simulink model "et_robocon_emer"  (R2014b)
settings: Solver=ode3  SolverMode=SingleTasking  StartTime=0.0  StopTime=10.0  RelTol=1e-3
undefined symbols (not defined in the file): balancerStates_Bus0, Batt, current_mode_status, current_task_operation_status, GYRO, Init_Bus0, K, lightCalib, PHI, R, RM, Th, TRACK_MODE_LIST, W
libraries: legonxtlib x27, ControllersFcns x5, simulink_extras x4, simulink x3, NXTFcns x2, gyro_calibration_algorithm_atomic_sub_chart_library x1, light_sensor_calibration_algorithm_atomic_sub_chart_library x1, plantNXT x1
(part 2 of 2)

== stateflow chart et_robocon_emer/Main Controller/normal_operation_modes.line_following_down ==
  state RampDownDir
    entry:
    StatusLCD(uint16(400));
    des_vel = single(0);
    desired_tail = single(0.0);
    BT_status_out = single(11);
    turningPWM = single(0);
    initFlags.theta = single(1);
    initFlags.gyroReset = single(1);
    Speak;
    during:
    normalizedLight = processLight(sensors.light,lightCalib);
    PWM.tail = tail_controller(sensors.theta_T, desired_tail);
    state Waiting
      entry:
      during:
      StatusLCD(uint16(400));
    state light = processLight(rawLight,lightCalib) [function]
    state cmd = lineTracker(desiredLight,light,trackingPower,battery) [function]
    state StandUp1
      entry:
      StatusLCD(uint16(401));
      initFlags.theta = single(1);
      initFlags.gyroReset = single(1);
    state cmd = balance_ctrl(balancerStates,desired_velocity,battery) [function]
    state Balancing
      state SeesawLogic [parallel]
        settings: executionOrder=2
        state MoveForwardSlowly
          entry:
          Speak;
          StatusLCD(uint16(402));
          des_vel = single(0.0);
          initFlags.theta = single(0);
          initFlags.gyroReset = single(0);
          storedphi = states.phi;
          tix = 1;
          des_vel = single(0.005);
          desired_phi = storedphi;
          thetaentry = states.balancerStates.theta;
          during:
          storedphi = storedphi+states.phi;
          tix = tix+1;
          turningPWM = lineTracker(single(-0.3), normalizedLight, single(1.5), sensors.battery)+...
          single(.5)*phiController(desired_phi,states.phi,sensors.battery);
        state StationnaryBalance
          entry:
          Speak;
          StatusLCD(uint16(403));
          storedphi = single(storedphi/tix);
          %StatusLCD(uint16(single(0.15)));
          des_vel = single(0.01);
          desired_phi = states.phi;
          during:
          des_vel = des_vel+single(0.001)
          turningPWM = lineTracker(single(-0.3), normalizedLight, single(1.5), sensors.battery)+...
          single(.5)*phiController(desired_phi,states.phi,sensors.battery);
          if des_vel > single(0.05)
          des_vel = single(0.05);
          end
        state constspeed
          entry: StatusLCD(uint16(404));
          during:
          turningPWM = phiController(desired_phi,states.phi,sensors.battery);
        state Ramps
          state Ramp2
            entry:
            thetaentry = states.balancerStates.theta;
            Speak;
            desired_phi = storedphi;
            %+single(0.5);
            %storedphi = states.phi;
            tix = 1;
            %Speak;
            StatusLCD(uint16(405));
            des_vel = single(0.03);
            %desired_phi = storedphi;
            during:
            %storedphi = storedphi +states.phi;
            %tix = tix+1;
            %des_vel = single(0.04);
            turningPWM = phiController(desired_phi,states.phi,sensors.battery);
            %turningPWM = lineTracker(single(-0.2),normalizedLight,single(1.5),sensors.battery)+...
            % single(.4)*phiController(desired_phi,states.phi,sensors.battery);
          state TurnLineTrackOn
            entry:
            StatusLCD(uint16(406));
            during:
            turningPWM = lineTracker(single(0.7),normalizedLight,single(1.5),sensors.battery)+...
            single(.5)*phiController(desired_phi,states.phi,sensors.battery);
          state Bridge
            entry:
            thetaentry = states.balancerStates.theta;
            Speak;
            StatusLCD(uint16(407));
            %storedphi = single(storedphi/tix);
            desired_phi  = storedphi;
            during:
            des_vel =single(0.04);
            turningPWM = phiController(desired_phi,states.phi,sensors.battery);
          state Ramp1
            entry:
            thetaentry = states.balancerStates.theta;
            des_vel= single(0.02);
            Speak;
            StatusLCD(uint16(408));
            during:
            during:
            turningPWM = lineTracker(single(0.7),normalizedLight,single(1.5),sensors.battery)+...
            single(.5)*phiController(desired_phi,states.phi,sensors.battery);
          state Land
            entry:
            des_vel= single(0.005);
            Speak;
            StatusLCD(uint16(409));
            during:
            turningPWM = phiController(desired_phi,states.phi,sensors.battery);
          (default) -> RampDownDir.Balancing.SeesawLogic.Ramps.Ramp2
          RampDownDir.Balancing.SeesawLogic.Ramps.Ramp2 -> TurnLineTrackOn : [states.balancerStates.theta>thetaentry + single(1*2*3.14) ]
          TurnLineTrackOn -> RampDownDir.Balancing.SeesawLogic.Ramps.Bridge : [states.balancerStates.theta>thetaentry + single(2*2*3.14) ]
          RampDownDir.Balancing.SeesawLogic.Ramps.Bridge -> RampDownDir.Balancing.SeesawLogic.Ramps.Ramp1 : [states.balancerStates.theta>thetaentry + single(1.57*2*3.14)]
          RampDownDir.Balancing.SeesawLogic.Ramps.Ramp1 -> Land : [states.balancerStates.theta> thetaentry+single(2.05*2*3.14)]
        state Ramp [commented out]
          state Ramp1 [commented out]
            entry:
            thetaentry = states.balancerStates.theta;
            desired_phi = states.phi;
            storedphi = states.phi;
            Speak;
            StatusLCD(uint16(3061));
            des_vel = single(0.08);
            tix = 0;
            during:
            storedphi = storedphi +states.phi;
            tix = tix+1;
            turningPWM = lineTracker(single(-0.15),normalizedLight,single(1),sensors.battery)
            %+...
            % phiController(desired_phi,states.phi,sensors.battery);
            %storedphi = states.phi; && states.balancerStates.psi_dot<single(-0.8)
          state Bridge [commented out]
            entry:
            thetaentry = states.balancerStates.theta;
            Speak;
            StatusLCD(uint16(3062));
            storedphi = single(storedphi/tix);
            desired_phi  = storedphi;
            during:
            des_vel =single(0.06);
            %turningPWM = lineTracker(single(-0.12),normalizedLight,single(1.3),sensors.battery)+...
            %   phiController(desired_phi,states.phi,sensors.battery);
            turningPWM = phiController(desired_phi,states.phi,sensors.battery);
          state Ramp2 [commented out]
            entry:
            thetaentry = states.balancerStates.theta;
            Speak;
            %Speak;
            StatusLCD(uint16(3063));
            des_vel = single(0.08);
            desired_phi = storedphi;
            during:
            %des_vel = single(0.04);
            %turningPWM = phiController(desired_phi,states.phi,sensors.battery);
            turningPWM = lineTracker(single(-0.15),normalizedLight,single(1.5),sensors.battery)+...
            single(.5)*phiController(desired_phi,states.phi,sensors.battery);
          state MtnTop [commented out]
            entry:
            Speak;
            thetaentry = states.balancerStates.theta;
            desired_phi = storedphi;
            StatusLCD(uint16(3064));
            des_vel = single(0.08);
            during:
            %turningPWM = lineTracker(single(-0.15),normalizedLight,single(1.2),sensors.battery)+...
            %    phiController(desired_phi,states.phi,sensors.battery);
            turningPWM = lineTracker(single(-0.15),normalizedLight,single(1.2),sensors.battery)+...
            single(0.5)*phiController(desired_phi,states.phi,sensors.battery);
            des_vel = single(0.001)+des_vel;
            if des_vel > single(0.1)
            des_vel = single(0.1);
            end
          state Slowdown [commented out]
            entry:
            Speak;
            StatusLCD(uint16(3065));
            during:
            turningPWM = lineTracker(single(-0.15),normalizedLight,single(1.2),sensors.battery)+...
            phiController(desired_phi,states.phi,sensors.battery)
            des_vel = des_vel - single(.0005);
          state Stop [commented out]
            entry:
            desired_phi = storedphi;
            %desiredangle = states.phi;
            Speak;
            StatusLCD(uint16(3066));
            StatusLCD(uint16(3064));
            des_vel = single(0.000);
          state Turn1 [commented out]
            entry:
            desired_phi = states.phi;
            %desiredangle = states.phi;
            Speak;
            StatusLCD(uint16(3067));
            des_vel = single(0.0005);
            during:
            turningPWM = phiController(desired_phi,states.phi,sensors.battery)
            desired_phi = desired_phi+single(.005);
          state STOP [commented out]
            entry: StatusLCD(uint16(3065));
            Speak;
            des_vel = single(0.00);
            desired_phi = states.phi;
            during:
            turningPWM = phiController(desired_phi,states.phi,sensors.battery);
          (default) -> RampDownDir.Balancing.SeesawLogic.Ramp.Ramp1 [commented out]
          RampDownDir.Balancing.SeesawLogic.Ramp.Ramp1 -> RampDownDir.Balancing.SeesawLogic.Ramp.Bridge [commented out] : [states.balancerStates.theta> thetaentry+single(2.05*2*3.14)]
          RampDownDir.Balancing.SeesawLogic.Ramp.Bridge -> RampDownDir.Balancing.SeesawLogic.Ramp.Ramp2 [commented out] : [states.balancerStates.theta>thetaentry + single(1.6*2*3.14)]
              | %[(states.balancerStates.theta> thetaentry+single(6*2*3.14)  && states.balancerStates.theta_dot>single(4.5)) || states.balancerStates.theta> thetaentry+single(10*2*3.14) ]
          RampDownDir.Balancing.SeesawLogic.Ramp.Ramp2 -> MtnTop [commented out] : [states.balancerStates.theta>thetaentry + single(2*2*3.14) && (states.balancerStates.psi < single(0) || states.balancerStates.psi_dot<single(-0.8))]
              | %[(states.balancerStates.theta> thetaentry+single(6.0*2*3.14) && states.balancerStates.theta_dot< -single(3.0)) || sensors.touch]
          MtnTop -> Slowdown [commented out] : [states.balancerStates.theta> thetaentry+single(0.95*2*3.14)]
          Slowdown -> Stop [commented out] : [des_vel<single(0)]
          Stop -> Turn1 [commented out] : after(2.5,sec)
          Turn1 -> STOP [commented out] : [states.phi > storedphi +single(3.14)] %3.5
          STOP -> ? [commented out] : after(1,sec)
        state CalibComplete [commented out]
          entry:
          StatusLCD(uint16(307));
          current_mode_status = OperationModeStatusEnum.SUCCESSFULLY_COMPLETED;
        (default) -> MoveForwardSlowly
        MoveForwardSlowly -> StationnaryBalance : after(2,sec)
        StationnaryBalance -> constspeed : [states.balancerStates.theta>thetaentry + single(0.7*2*3.14) ]
        constspeed -> Ramps : [states.balancerStates.theta_dot>single(5) || states.balancerStates.psi_dot<single(-0.8)]
        (default) -> Ramp [commented out] : [sensors.touch || states.balancerStates.theta_dot<single(0.8)]
      state After [parallel]
        during:
        forwardPWM = balance_ctrl(states.balancerStates, des_vel ,sensors.battery)
        PWM.left = forwardPWM + turningPWM;
        PWM.right = forwardPWM - turningPWM;
        settings: executionOrder=1
    Waiting -> StandUp1 : [sensors.touch]
    (default) -> Waiting
    StandUp1 -> Balancing
  data: rawLight function_input single size=1; lightCalib function_input Bus: Light_Bus size=1; light function_output; cmd function_output single size=1; desiredLight function_input single size=1; light function_input single size=1; trackingPower function_input single size=1; battery function_input double size=1; balancerStates function_input Bus: Balancer_States_Bus size=1; desired_velocity function_input single size=1; battery function_input double size=1; cmd function_output single size=1; states input; sensors input Bus: Sensors_Bus size=1; PWM output Bus: PWM_bus size=1; current_mode_status data_store_memory; lightCalib data_store_memory; BT_status_out output single size=1; desired_tail local; turningPWM local; normalizedLight local; forwardPWM local; des_vel local; desired_phi local; desiredangle local; storedphi local; thetaentry local; tix local; initFlags output Bus: Init_Bus size=1; des_phi local

== stateflow chart et_robocon_emer/State Estimation/StateEstimation/Reset Subsystem ==
  state CheckForReset
    bind: doProcess;
    entry: doProcess;
    during: doProcess;
  (default) -> CheckForReset
  CheckForReset -> CheckForReset : [init_flag == 1]
  data: init_flag input
  events: doProcess output FUNCTION_CALL_EVENT

== stateflow chart et_robocon_emer/Main Controller ==
  state emergency_stop
    entry:
    DebugFlag = uint16(99);
    StatusLCD(DebugFlag);
  state normal_operation_modes
    state gyro_calibration_mode
    state light_calibration_up
    state NXT_Up_Down
    state line_following_down
    state WeShouldNotBeHere
    (default) -> (junction 12) : {
        | current_mode_status = OperationModeStatusEnum.IN_PROGRESS;
        | }
    (junction 12) -> gyro_calibration_mode [order 1] : [  current_mode == OperationModeEnum.GYRO_CALIBRATION ]
    (junction 12) -> (junction 13) [order 2]
    (junction 13) -> light_calibration_up [order 1] : [ current_mode == OperationModeEnum.LIGHT_CALIBRATION_UP ]
    (junction 13) -> (junction 144) [order 2]
    (junction 144) -> (junction 14)
    (junction 14) -> NXT_Up_Down [order 1] : [ current_mode == OperationModeEnum.LINE_TRACKING]
    (junction 14) -> (junction 19) [order 2]
    (junction 19) -> line_following_down [order 1] : [ current_mode == OperationModeEnum.SEE_SAW_MARIO]
    (junction 19) -> (junction 99) [order 2]
    (junction 99) -> WeShouldNotBeHere
  (default) -> (junction 38) : {initFlags = Init_Bus0;BT_status_out = single(0)}
  (junction 37) -> (junction 38)
  (junction 43) -> (junction 37)
  (junction 38) -> (junction 39) : { current_mode_index = uint8( 0 ); }
  (junction 40) -> (junction 39)
  emergency_stop -> (junction 40)
  (junction 39) -> (junction 41) : {
      | current_mode_status = OperationModeStatusEnum.NOT_STARTED;
      | }
  normal_operation_modes -> (junction 40) [order 2] : [ current_mode_status == OperationModeStatusEnum.SUCCESSFULLY_COMPLETED ]
  normal_operation_modes -> emergency_stop [order 1] : [ sensors.ok_button ]
      | {current_mode_status = OperationModeStatusEnum.ABORTED;}
  (junction 42) -> (junction 41)
  (junction 41) -> (junction 44) : { current_mode_index = current_mode_index + uint8( 1 ); }
  (junction 47) -> (junction 42)
  (junction 44) -> (junction 43) [order 1] : [ numel( TRACK_MODE_LIST ) < current_mode_index ]
      | % If the "current_mode_index" has exceeded the number
      | % of elements in the list, it should "wrap" back to the start.
  (junction 44) -> (junction 45) [order 2]
  (junction 45) -> (junction 46) : {
      | current_mode = TRACK_MODE_LIST( current_mode_index );
      | }
  (junction 46) -> (junction 47) [order 1] : [  current_mode == OperationModeEnum.SKIP ]
  (junction 46) -> normal_operation_modes [order 2]
  data: PWM output Bus: PWM_bus size=1; TRACK_MODE_LIST parameter Enum: OperationModeEnum; current_mode_index local uint8; current_mode data_store_memory; states input Bus: States_Bus size=1; current_mode_status data_store_memory; sensors input Bus: Sensors_Bus size=1; lightCalib data_store_memory; BT_status_out output single size=1; initFlags output Bus: Init_Bus size=1; Init_Bus0 parameter Bus: Init_Bus size=1; balancerStates_Bus0 parameter Bus: Balancer_States_Bus size=1; phi_des data_store_memory size=1; DebugFlag output uint16 size=1; normalizedLight output single size=1

== stateflow chart et_robocon_emer/Main Controller/normal_operation_modes.NXT_Up_Down ==
  state RampUpDir
    entry:
    des_vel = single(0.0);
    desired_tail = single(0.0);
    %BT_status_out = single(11);
    Speak;
    during:
    normalizedLight = processLight(sensors.light,lightCalib);
    PWM.tail = tail_controller(sensors.theta_T, desired_tail);
    state Waiting
      during:
      DebugFlag = uint16(300);
      StatusLCD(DebugFlag);
    state cmd = balance_ctrl(balancerStates,desired_velocity,battery) [function]
    state light = processLight(rawLight,lightCalib) [function]
    state StandUp
      entry:
      DebugFlag = uint16(301);
      StatusLCD(DebugFlag);
      initFlags.theta = single(1);
      initFlags.gyroReset = single(1);
    state cmd = lineTracker(desiredLight,light,trackingPower,battery) [function]
    state Balancing
      state SeesawLogic [parallel]
        settings: executionOrder=1
        state MoveForwardSlowly
          entry:
          Speak;
          DebugFlag = uint16(302);
          StatusLCD(DebugFlag);
          initFlags.theta = single(0);
          initFlags.gyroReset = single(0);
          des_vel = single(0.0005);
          %desired_states = balancerStates_Bus0;
          %turningPWM = single(0);
        state StationaryBalance
          entry:
          Speak;
          DebugFlag = uint16(303);
          StatusLCD(DebugFlag);
          %StatusLCD(uint16(single(0.15)));
          des_vel = single(0.0005);
          desired_phi = states.phi;
          exit:
          turningPWM =     phiController(desired_phi,states.phi,sensors.battery);
          %lineTracker(single(-0.1), normalizedLight, single(1.3), sensors.battery);
        state SpeedUp
          entry:
          Speak;
          DebugFlag = uint16(304);
          StatusLCD(DebugFlag);
          thetaentry = states.balancerStates.theta;
          %StatusLCD(uint16(304));
          %des_vel = single(0.001);
          during:
          des_vel = single(0.02); % min(0.02,des_vel+single(0.005));
          turningPWM = lineTracker(single(-0.12), normalizedLight, single(1.2), sensors.battery);
        state ConstantSpeed
          entry:
          Speak;
          DebugFlag = uint16(305);
          StatusLCD(DebugFlag);
          during:
          %turningPWM = lineTracker(single(-0.15), normalizedLight, single(1.2), sensors.battery);
          turningPWM = lineTracker(single(-0.19), normalizedLight, single(1.2), sensors.battery);
          state RecordPhi
            entry:
            storedphi = states.phi;
            tix = 1;
            during:
            storedphi = storedphi+states.phi;
            tix = tix+1;
          ConstantSpeed -> RecordPhi [order 1]
        state RampUp
          state Ramp1_Up
            entry:
            desired_phi = single(storedphi/tix);
            thetaentry = states.balancerStates.theta;
            %desired_phi = states.phi;
            storedphi = states.phi;
            Speak;
            DebugFlag = uint16(306);
            StatusLCD(DebugFlag);
            des_vel = single(0.08);
            tix =1;
            during:
            storedphi = storedphi +states.phi;
            tix = tix+1;
            turningPWM = lineTracker(single(-0.06),normalizedLight,single(1),sensors.battery)+...
            single(0.5)*phiController(desired_phi,states.phi,sensors.battery);
            %+...
            % phiController(desired_phi,states.phi,sensors.battery);
            %storedphi = states.phi; && states.balancerStates.psi_dot<single(-0.8)
          state Bridge_Up
            entry:
            thetaentry = states.balancerStates.theta;
            Speak;
            DebugFlag = uint16(307);
            StatusLCD(DebugFlag);
            storedphi = single(storedphi/tix);
            desired_phi  = storedphi;
            during:
            des_vel =single(0.06);
            %turningPWM = lineTracker(single(-0.12),normalizedLight,single(1.3),sensors.battery)+...
            %   phiController(desired_phi,states.phi,sensors.battery);
            turningPWM = phiController(desired_phi,states.phi,sensors.battery);
          state Ramp2_Up
            entry:
            thetaentry = states.balancerStates.theta;
            Speak;
            storedphi2 = states.phi;
            tix2 = 1;
            %Speak;
            DebugFlag = uint16(308);
            StatusLCD(DebugFlag);
            des_vel = single(0.07);
            desired_phi = storedphi;
            during:
            %des_vel = single(0.04);
            %turningPWM = phiController(desired_phi,states.phi,sensors.battery);
            turningPWM = lineTracker(single(-0.07),normalizedLight,single(1.5),sensors.battery)+...
            single(.4)*phiController(desired_phi,states.phi,sensors.battery);
            storedphi2 = storedphi2+states.phi;
            tix2 = tix2+1;
            if states.balancerStates.theta>thetaentry + single(1.7*2*3.14)
            turningPWM= single(0)*lineTracker(single(-0.08),normalizedLight,single(1.5),sensors.battery)+...
            single(1)*phiController(desired_phi,states.phi,sensors.battery);
            end
          state MtnTop_Up
            entry:
            Speak;
            storedphi2 = single(storedphi2/tix2);
            %thetaentry = states.balancerStates.theta;
            desired_phi = storedphi;
            DebugFlag = uint16(309);
            StatusLCD(DebugFlag);
            des_vel = single(0.08);
            during:
            %turningPWM = lineTracker(single(-0.15),normalizedLight,single(1.2),sensors.battery)+...
            %    phiController(desired_phi,states.phi,sensors.battery);
            turningPWM = single(0)*lineTracker(single(0.1),normalizedLight,single(1.6),sensors.battery)+...
            single(1.0)*phiController(desired_phi,states.phi,sensors.battery);
            %des_vel = single(0.001)+des_vel;
            %if des_vel > single(0.1)
            %    des_vel = single(0.1);
            %end
          state Slowdown_Up
            entry:
            Speak;
            DebugFlag = uint16(310);
            StatusLCD(DebugFlag);
            during:
            turningPWM = lineTracker(single(0.3),normalizedLight,single(1.2),sensors.battery)+...
            single(0.25)*phiController(desired_phi,states.phi,sensors.battery)
            des_vel = des_vel - single(.0001); %0.1*phi
            if des_vel<=single(0.04)
            des_vel = single(0.04);
            end
          state Turn_Backwards_Up
            entry:
            desired_phi = states.phi;
            %desiredangle = states.phi;
            Speak;
            DebugFlag = uint16(311);
            StatusLCD(DebugFlag);
            des_vel = single(0.01);
            during:
            turningPWM = phiController(desired_phi,states.phi,sensors.battery);
            desired_phi = desired_phi+single(.01);
          state Stop_Up
            entry:
            desired_phi = states.phi;
            thetaentry = states.balancerStates.theta;
            BT_status_out = single(1);
            DebugFlag = uint16(312);
            StatusLCD(DebugFlag);
            Speak;
            des_vel = single(0.03);
            %desired_phi = states.phi;
            during:
            turningPWM = phiController(desired_phi,states.phi,sensors.battery);
          (default) -> Ramp1_Up
          Ramp1_Up -> Bridge_Up : [states.balancerStates.theta> thetaentry+single(2.05*2*3.14)]
          Bridge_Up -> Ramp2_Up : [states.balancerStates.theta>thetaentry + single(1.57*2*3.14)]
              | %[(states.balancerStates.theta> thetaentry+single(6*2*3.14)  && states.balancerStates.theta_dot>single(4.5)) || states.balancerStates.theta> thetaentry+single(10*2*3.14) ]
          Ramp2_Up -> MtnTop_Up : [states.balancerStates.theta>thetaentry + single(2.0*2*3.14) && (states.balancerStates.psi < single(0) || states.balancerStates.psi_dot<single(-0.5))]
              | %[(states.balancerStates.theta> thetaentry+single(6.0*2*3.14) && states.balancerStates.theta_dot< -single(3.0)) || sensors.touch]
          MtnTop_Up -> Slowdown_Up : [states.balancerStates.theta> thetaentry+single(3.5*2*3.14)]
          Slowdown_Up -> Turn_Backwards_Up : [states.balancerStates.theta> thetaentry+single(4.1*2*3.14) ]
          Turn_Backwards_Up -> Stop_Up : [states.phi > storedphi +single(3.05)] %3.5
        state MoveForwardSlowly_Down
          entry:
          Speak;
          DebugFlag = uint16(402);
          StatusLCD(DebugFlag);
          %des_vel = single(0.0);
          %initFlags.theta = single(0);
          %initFlags.gyroReset = single(0);
          %storedphi = states.phi;
          %tix = 1;
          %desired_phi = storedphi+single(3.17);
          des_vel = single(0.005);
          %desired_phi = storedphi;
          thetaentry = states.balancerStates.theta;
          during:
          des_vel = des_vel+0.001
          %storedphi = storedphi+states.phi;
          %tix = tix+1;
          turningPWM = lineTracker(single(0.3), normalizedLight, single(1.5), sensors.battery);
          if des_vel > single(0.03)
          des_vel = single(0.03);
          end
          %single(.9)*phiController(desired_phi,states.phi,sensors.battery);
        state constspeed_Down
          entry:
          Speak;
          des_vel = single(0.04);
          %desired_phi = storedphi+single(3.14);
          desired_phi = storedphi+ single(3.44);
          DebugFlag = uint16(404);
          StatusLCD(DebugFlag);
          during:
          turningPWM = phiController(desired_phi,states.phi,sensors.battery);
        state RampDown
          state Ramp2_Down
            entry:
            thetaentry = states.balancerStates.theta;
            Speak;
            %desired_phi = storedphi2+ single(3.23);
            %desired_phi = storedphi;
            %+single(0.5);
            %storedphi = states.phi;
            tix = 1;
            %Speak;
            DebugFlag = uint16(405);
            StatusLCD(DebugFlag);
            des_vel = single(0.04); %0.03
            %desired_phi = storedphi;
            during:
            %storedphi = storedphi +states.phi;
            %tix = tix+1;
            %des_vel = single(0.04);
            turningPWM = phiController(desired_phi,states.phi,sensors.battery);
            %turningPWM = lineTracker(single(-0.2),normalizedLight,single(1.5),sensors.battery)+...
            % single(.4)*phiController(desired_phi,states.phi,sensors.battery);
          state TurnLineTrackOn_Down
            entry:
            des_vel = single(0.05);
            DebugFlag = uint16(406);
            StatusLCD(DebugFlag);
            during:
            turningPWM = lineTracker(single(0.7),normalizedLight,single(1.5),sensors.battery)+...
            single(.5)*phiController(desired_phi,states.phi,sensors.battery);
          state Bridge_Down
            entry:
            initFlags.theta = single(1);
            initFlags.theta = single(0);
            thetaentry = states.balancerStates.theta;
            Speak;
            DebugFlag = uint16(407);
            StatusLCD(DebugFlag);
            %storedphi = single(storedphi/tix);
            %desired_phi  = storedphi;
            during:
            des_vel =single(0.03);
            turningPWM = phiController(desired_phi,states.phi,sensors.battery);
          state Ramp1_Down
            entry:
            thetaentry = states.balancerStates.theta;
            des_vel= single(0.03);
            Speak;
            DebugFlag = uint16(408);
            StatusLCD(DebugFlag);
            during:
            turningPWM = lineTracker(single(0.7),normalizedLight,single(1.5),sensors.battery)+...
            single(.5)*phiController(desired_phi,states.phi,sensors.battery);
            if states.balancerStates.theta> thetaentry+single(1*2*3.14)
            des_vel= single(0.06);
            end
          state GroundGoForward
            entry:
            BT_status_out = single(2);
            des_vel= single(0.0001);
            Speak;
            DebugFlag = uint16(410);
            StatusLCD(DebugFlag);
            during:
            turningPWM = phiController(desired_phi,states.phi,sensors.battery);
          state Ground
            entry:
            thetaentry = states.balancerStates.theta;
            des_vel= single(0.05);
            Speak;
            DebugFlag = uint16(409);
            StatusLCD(DebugFlag);
            during:
            turningPWM = phiController(desired_phi,states.phi,sensors.battery);
          (default) -> Ramp2_Down
          Ramp2_Down -> TurnLineTrackOn_Down : [states.balancerStates.theta>thetaentry + single(1*2*3.14) ]
          TurnLineTrackOn_Down -> Bridge_Down : [states.balancerStates.theta>thetaentry + single(2*2*3.14) ]
          Bridge_Down -> Ramp1_Down : [states.balancerStates.theta>thetaentry + single(1.57*2*3.14)]
          Ramp1_Down -> Ground : [states.balancerStates.theta> thetaentry+single(2.15*2*3.14) && states.balancerStates.psi_dot<single(-0.8) ]
          Ground -> GroundGoForward : [states.balancerStates.theta> thetaentry+single(0.35*2*3.14)]
        state Rotate_Right
          entry:
          desired_phi = states.phi;
          %desiredangle = states.phi;
          Speak;
          DebugFlag = uint16(501);
          StatusLCD(DebugFlag);
          des_vel = single(0.001);
          during:
          turningPWM = phiController(desired_phi,states.phi,sensors.battery);
          desired_phi = desired_phi-single(.01);
        state CalibComplete [commented out]
          entry:
          StatusLCD(uint16(307));
          current_mode_status = OperationModeStatusEnum.SUCCESSFULLY_COMPLETED;
        state GoStraight
          entry:
          desired_phi = states.phi;
          thetaentry = states.balancerStates.theta;
          Speak;
          DebugFlag = uint16(502);
          StatusLCD(DebugFlag);
          des_vel = single(0.05);
          during:
          turningPWM = phiController(desired_phi,states.phi,sensors.battery);
        state GoTowardsZone
          entry:
          Speak;
          DebugFlag = uint16(503);
          StatusLCD(DebugFlag);
          during:
          turningPWM = phiController(desired_phi,states.phi,sensors.battery);
          desired_phi = desired_phi-single(0.001);
        state RotateInPlace
          entry:
          Speak;
          DebugFlag = uint16(505);
          StatusLCD(DebugFlag);
          desired_phi = states.phi;
          during:
          des_vel = max(des_vel-single(0.001),0);
          desired_phi = desired_phi+single(0.005);
          turningPWM = phiController(desired_phi,states.phi,sensors.battery);
          if storedphi+single(2*6.4)<states.phi
          turningPWM = single(0);
          %des_vel = single(0.002);
          end
        state GoTowardsZone2
          entry:
          Speak;
          DebugFlag = uint16(504);
          StatusLCD(DebugFlag);
          thetaentry = states.balancerStates.theta;
          des_vel = single(0.04);
          Speak;
          DebugFlag = uint16(504);
          StatusLCD(DebugFlag);
          during:
          turningPWM = phiController(desired_phi,states.phi,sensors.battery);
        (default) -> MoveForwardSlowly
        MoveForwardSlowly -> StationaryBalance : after(2,sec)
        StationaryBalance -> SpeedUp : after(0.08,sec)
        SpeedUp -> ConstantSpeed : [states.balancerStates.theta> thetaentry+ single(2*3.14)] %0.15
        ConstantSpeed -> RampUp [order 1] : [states.balancerStates.theta_dot<single(0.6)] %states.phi>single(3) && states.balancerStates.theta_dot<single(0.8)
        MoveForwardSlowly_Down -> constspeed_Down : [states.balancerStates.theta>thetaentry + single(0.65*2*3.14) ]
        constspeed_Down -> RampDown : [states.balancerStates.theta_dot>single(5) || states.balancerStates.psi_dot<single(-0.8)]
        Rotate_Right -> GoStraight : [states.phi< storedphi+single(1.45)]
        GoStraight -> GoTowardsZone : [states.balancerStates.theta>thetaentry+ single(2.0*2*3.14)]
        GoTowardsZone -> GoTowardsZone2 : [states.phi<storedphi+single(0.7)]
        GoTowardsZone2 -> RotateInPlace : [states.balancerStates.theta>thetaentry+ single(2.0*2*3.14)]
        GroundGoForward -> Rotate_Right : after(2,sec)
        Stop_Up -> MoveForwardSlowly_Down : [states.balancerStates.theta> thetaentry+ single(0.45*2*3.14)] %0.15
      state After [parallel]
        entry:
        fall_detected = false;
        during:
        if (single(1.1)<abs(states.balancerStates.psi))
        DebugFlag = uint16(999);
        StatusLCD(DebugFlag);
        BT_status_out = single(99);
        PWM.left = single(0);
        PWM.right = single(0);
        fall_detected = true;
        else
        if (~fall_detected)
        forwardPWM = balance_ctrl(states.balancerStates, des_vel ,sensors.battery);
        PWM.left = forwardPWM + turningPWM;
        PWM.right = forwardPWM - turningPWM;
        end
        end
        settings: executionOrder=2
    (default) -> Waiting
    Waiting -> StandUp : [sensors.touch]
    StandUp -> Balancing
  data: balancerStates function_input Bus: Balancer_States_Bus size=1; desired_velocity function_input single size=1; battery function_input double size=1; cmd function_output single size=1; rawLight function_input single size=1; lightCalib function_input Bus: Light_Bus size=1; light function_output; cmd function_output single size=1; desiredLight function_input single size=1; light function_input single size=1; trackingPower function_input single size=1; battery function_input double size=1; sensors input Bus: Sensors_Bus size=1; lightCalib data_store_memory; current_task_operation_status data_store_memory; PWM output Bus: PWM_bus size=1; initFlags output Bus: Init_Bus size=1; BT_status_out output; desired_tail local; balancerStates_Bus0 parameter; turningPWM local; states input; normalizedLight output single size=1; forwardPWM local; des_vel local; desired_phi local; desiredangle local; storedphi local; thetaentry local; tix local; DebugFlag output uint16 size=1; tix2 local; storedphi2 local; fall_detected local boolean
